simulink model "FBR_Buck_Sim_Final"  (R2022b)
settings: Solver=VariableStepAuto  StartTime=0.0  StopTime=0.04  RelTol=1e-3
libraries: spsDiodeLib x7, spsMeanLib x6, spsACVoltageSourceLib x3, spsCurrentMeasurementLib x2, spsSeriesRLCBranchLib x2, spsVoltageMeasurementLib x2, spsDCVoltageSourceLib x1, spsIGBTLib x1, eePwmGenerator x1, sps_lib x1
settings Model: Creator=Mekatrona  LastModifiedBy=Mekatrona

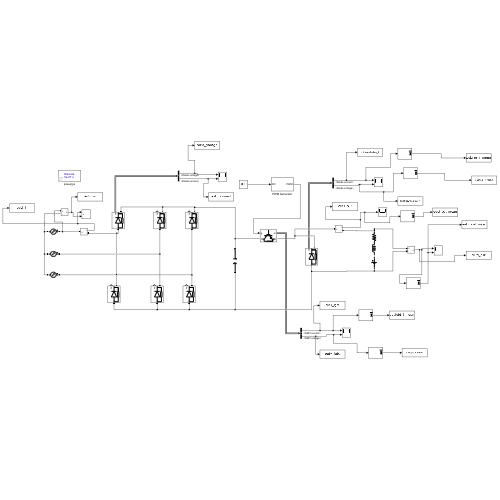
[thumbnail: Simulink's stored preview of the top-level diagram]
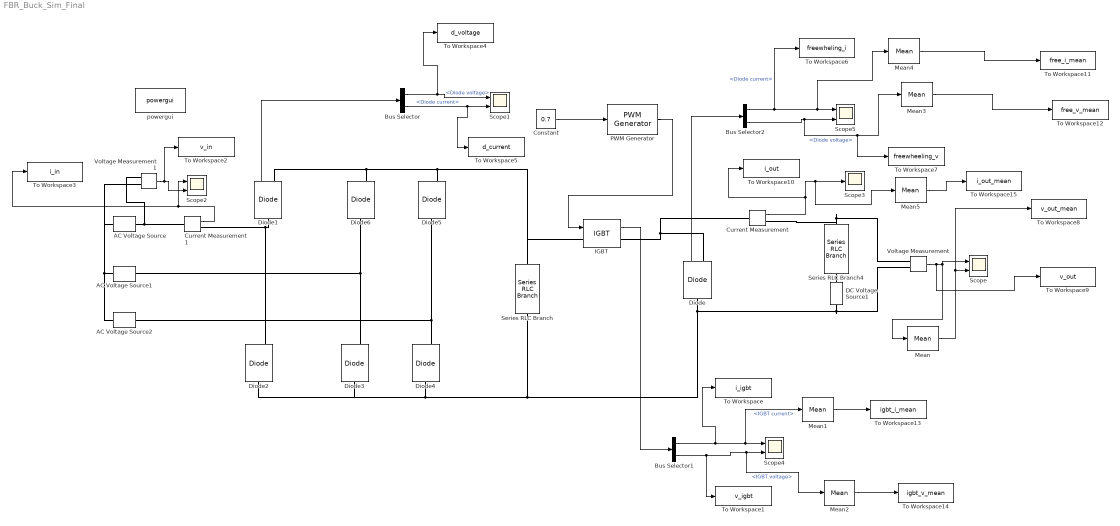
== system FBR_Buck_Sim_Final ==
  AC Voltage Source : spsACVoltageSourceLib/AC Voltage Source  Amplitude=160  Phase=0  Frequency=50  SampleTime=0  Measurements=None  BusType=swing  Pref=10e3  Qref=0  Qmin=-inf  Qmax=+inf
  AC Voltage Source1 : spsACVoltageSourceLib/AC Voltage Source  Amplitude=160  Phase=120  Frequency=50  SampleTime=0  Measurements=None  BusType=swing  Pref=10e3  Qref=0  Qmin=-inf  Qmax=+inf
  AC Voltage Source2 : spsACVoltageSourceLib/AC Voltage Source  Amplitude=160  Phase=240  Frequency=50  SampleTime=0  Measurements=None  BusType=swing  Pref=10e3  Qref=0  Qmin=-inf  Qmax=+inf
  Bus Selector : BusSelector  OutputSignals=Diode voltage,Diode current
  Bus Selector1 : BusSelector  OutputSignals=IGBT current,IGBT voltage
  Bus Selector2 : BusSelector  OutputSignals=Diode current,Diode voltage
  Constant : Constant  Value=0.7
  Current Measurement : spsCurrentMeasurementLib/Current Measurement  PhasorSimulation=off  OutputType=Complex  PSBequivalent=0
  Current Measurement1 : spsCurrentMeasurementLib/Current Measurement  PhasorSimulation=off  OutputType=Complex  PSBequivalent=0
  DC Voltage Source1 : spsDCVoltageSourceLib/DC Voltage Source  Amplitude=172  Measurements=None
  Diode : spsDiodeLib/Diode  Ron=0.001  Lon=0  Vf=0.8  IC=0  UseSnubber=0  Rs=500  Cs=250e-9  Measurements=on
  Diode{1..6} (6 alike) : spsDiodeLib/Diode  Ron=0.001  Lon=0  Vf=0.8  IC=0  UseSnubber=0  Rs=1e6  Cs=1e-9  Measurements=on
  IGBT : spsIGBTLib/IGBT  Ron=0.001  Lon=0  Vf=1  Tf=1e-6  Tt=2e-6  IC=0  Rs=1e5  Cs=inf  Measurements=on
  Mean{,1..5} (6 alike) : spsMeanLib/Mean  Freq=1000  Vinit=0  Ts=0
  PWM Generator : eePwmGenerator/PWM Generator  CarrCount=Up  Tper=1e-3  Tdelay=0  Ts=0
  Scope{,1..2,4..5} (5 alike) : Scope  NumInputPorts=2
  Scope3 : Scope
  Series RLC Branch : spsSeriesRLCBranchLib/Series RLC Branch  LConnTagsString=__new0  RConnTagsString=__new0  BranchType=C  Resistance=1  Inductance=1e-3  SetiL0=off  InitialCurrent=0  Capacitance=47e-6  Setx0=off  InitialVoltage=0  Measurements=None
  Series RLC Branch4 : spsSeriesRLCBranchLib/Series RLC Branch  LConnTagsString=__new0  RConnTagsString=__new0  BranchType=RL  Resistance=0.8  Inductance=12.5e-3  SetiL0=off  InitialCurrent=0  Capacitance=1e-6  Setx0=off  InitialVoltage=0  Measurements=None
  To Workspace : ToWorkspace  VariableName=i_igbt  SaveFormat=Timeseries  SampleTime=-1
  To Workspace1 : ToWorkspace  VariableName=v_igbt  SaveFormat=Timeseries  SampleTime=-1
  To Workspace10 : ToWorkspace  VariableName=i_out  SaveFormat=Timeseries  SampleTime=-1
  To Workspace11 : ToWorkspace  VariableName=free_i_mean  SaveFormat=Timeseries  SampleTime=-1
  To Workspace12 : ToWorkspace  VariableName=free_v_mean  SaveFormat=Timeseries  SampleTime=-1
  To Workspace13 : ToWorkspace  VariableName=igbt_i_mean  SaveFormat=Timeseries  SampleTime=-1
  To Workspace14 : ToWorkspace  VariableName=igbt_v_mean  SaveFormat=Timeseries  SampleTime=-1
  To Workspace15 : ToWorkspace  VariableName=i_out_mean  SaveFormat=Timeseries  SampleTime=-1
  To Workspace2 : ToWorkspace  VariableName=v_in  SaveFormat=Timeseries  SampleTime=-1
  To Workspace3 : ToWorkspace  VariableName=i_in  SaveFormat=Timeseries  SampleTime=-1
  To Workspace4 : ToWorkspace  VariableName=d_voltage  SaveFormat=Timeseries  SampleTime=-1
  To Workspace5 : ToWorkspace  VariableName=d_current  SaveFormat=Timeseries  SampleTime=-1
  To Workspace6 : ToWorkspace  VariableName=freewheling_i  SaveFormat=Timeseries  SampleTime=-1
  To Workspace7 : ToWorkspace  VariableName=freewheeling_v  SaveFormat=Timeseries  SampleTime=-1
  To Workspace8 : ToWorkspace  VariableName=v_out_mean  SaveFormat=Timeseries  SampleTime=-1
  To Workspace9 : ToWorkspace  VariableName=v_out  SaveFormat=Timeseries  SampleTime=-1
  Voltage Measurement : spsVoltageMeasurementLib/Voltage Measurement  PhasorSimulation=off  OutputType=Complex  PSBequivalent=0
  Voltage Measurement1 : spsVoltageMeasurementLib/Voltage Measurement  PhasorSimulation=off  OutputType=Complex  PSBequivalent=0
  powergui : sps_lib/powergui  Priority=1  SimulationMode=Discrete  SampleTime=5e-7  frequency=60  Iterations=50  frequencyindice=50  Pbase=100e6  ErrMax=1e-4  UnitsV=kV  UnitsW=MW  buscounter=0  FunctionMessages=off  echomessages=off  EnableUseOfTLC=off  CurrentSourceSwitches=off  DisableSnubberDevices=off  DisableRonSwitches=off  DisableVfSwitches=off  DisplayEquations=off  AutomaticDiscreteSolvers=off  SolverType=Tustin/Backward Euler (TBE)  Interpol=off  ExternalGateDelay=off  methode=off  Ts=100  x0status=blocks  SPID=on  SwTol=0  HookPort=off  NonlinearTolerance=1e-4  nMaxIteration=100  ContinueOnMaxIteration=off  RestoreLinks=warning  ResistiveCurrentMeasurement=off  Frange=[0:2:500]  Ylog=off  Xlog=on  ShowGrid=off  save=off  variable=ZData  structure=0  ZoomFFT=off  StartTime=0.0  cycles=1  DisplayStyle=1  fundamental=60  FreqAxis=off  MaxFrequency=1000  frequencyindicesteady=1  RmsSteady=1  display=off
  wires:
  Bus Selector/2 -> To Workspace5/1, Scope1/2  "<Diode current>"
  Voltage Measurement1/1 -> To Workspace2/1, Scope2/2
  Current Measurement1/1 -> To Workspace3/1, Scope2/1
  Diode1/1 -> Bus Selector/1
  Bus Selector/1 -> To Workspace4/1, Scope1/1  "<Diode voltage>"
  PWM Generator/1 -> IGBT/1
  Constant/1 -> PWM Generator/1
  Mean/1 -> To Workspace8/1, Scope/2
  Voltage Measurement/1 -> To Workspace9/1, Mean/1, Scope/1
  Current Measurement/1 -> To Workspace10/1, Mean5/1, Scope3/1
  IGBT/1 -> Bus Selector1/1
  Bus Selector1/1 -> To Workspace/1, Mean1/1, Scope4/1  "<IGBT current>"
  Bus Selector1/2 -> To Workspace1/1, Mean2/1, Scope4/2  "<IGBT voltage>"
  Bus Selector2/2 -> Mean3/1, To Workspace7/1, Scope5/2  "<Diode voltage>"
  Bus Selector2/1 -> To Workspace6/1, Mean4/1, Scope5/1  "<Diode current>"
  Diode/1 -> Bus Selector2/1
  Mean4/1 -> To Workspace11/1
  Mean3/1 -> To Workspace12/1
  Mean1/1 -> To Workspace13/1
  Mean2/1 -> To Workspace14/1
  Mean5/1 -> To Workspace15/1
  connections:
  AC Voltage Source1/LConn1 -- AC Voltage Source2/LConn1 -- AC Voltage Source/LConn1 -- Voltage Measurement1/LConn2
  Diode5/RConn1 -- IGBT/LConn1 -- Series RLC Branch/LConn1 -- Diode6/RConn1 -- Diode1/RConn1
  Voltage Measurement/LConn2 -- DC Voltage Source1/LConn1 -- Series RLC Branch/RConn1 -- Diode4/LConn1 -- Diode2/LConn1 -- Diode3/LConn1 -- Diode/LConn1
  Diode6/LConn1 -- AC Voltage Source1/RConn1 -- Diode3/RConn1
  Diode5/LConn1 -- AC Voltage Source2/RConn1 -- Diode4/RConn1
  Current Measurement1/RConn1 -- Diode2/RConn1 -- Diode1/LConn1
  AC Voltage Source/RConn1 -- Current Measurement1/LConn1 -- Voltage Measurement1/LConn1
  Diode/RConn1 -- IGBT/RConn1 -- Current Measurement/LConn1
  Series RLC Branch4/LConn1 -- Current Measurement/RConn1 -- Voltage Measurement/LConn1
  DC Voltage Source1/RConn1 -- Series RLC Branch4/RConn1
